simulink model "linearized_coupled_model"  (R2016b)
settings: Solver=VariableStepAuto  StartTime=0.0  StopTime=10.0  RelTol=1e-3
values from neighbouring files (symbols this model uses):
  A = simplify(A)    [symbolic_rotor.m]
  B_here = B_dbth    [riccati_controller_linear.m]
  C = [0,0,0,-L*mg*cos(beta)*beta_dot;0,0,0,L*mg*sin(beta)*beta_dot;0,0,0,0;0,0,0,0]    [disturbance_compensation_nonlinear_test.m]    (also in symbolic_rotor.m = [1,0,0,0, 0,0,0,0; uav_grasp_opt.m = [0,0,L*mg*sin(theta)*theta_dot;0,0,L*mg*cos(theta)*theta_dot; uav_grasp_opt_var_mass.m)
  K = diag([512,9,16])    [decoupling_falb_wolovich.m]
  V = inv(C*((B_here*K-A)\B_here))    [riccati_controller_linear.m]
  x0 = zeros(8,1)    [decoupling_falb_wolovich.m]    (also in disturbance_compensation.m; disturbance_compensation_nonlinear_test.m = [0;0;0;pi/2;0;0;0;0]; riccati_controller_linear.m; symbolic_rotor.m)
settings Model: Creator=Administrator  LastModifiedBy=Administrator

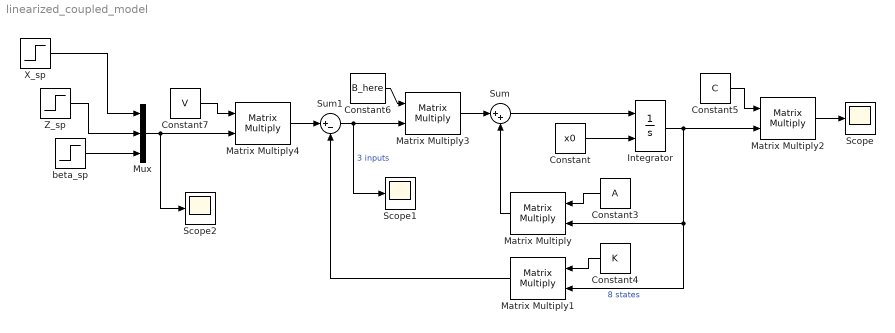
== system linearized_coupled_model ==
  Constant : Constant  Value=x0
  Constant3 : Constant  Value=A
  Constant4 : Constant  Value=K
  Constant5 : Constant  Value=C
  Constant6 : Constant  Value=B_here
  Constant7 : Constant  Value=V
  Integrator : Integrator  InitialConditionSource=external
  Matrix Multiply{,1..4} (5 alike) : Product  Multiplication=Matrix(*)
  Mux : Mux  Inputs=3
  Scope : Scope
  Scope1 : Scope
  Scope2 : Scope
  Sum : Sum  Inputs=|++
  Sum1 : Sum  Inputs=|+-
  X_sp : Step  SampleTime=0  VectorParams1D=off
  Z_sp : Step  SampleTime=0  VectorParams1D=off
  beta_sp : Step  Time=6  After=0.3  SampleTime=0  VectorParams1D=off
  wires:
  Constant/1 -> Integrator/2
  Sum/1 -> Integrator/1
  Integrator/1 -> Matrix Multiply1/2, Matrix Multiply/2, Matrix Multiply2/2  "8 states"
  Matrix Multiply/1 -> Sum/2
  Matrix Multiply3/1 -> Sum/1
  Matrix Multiply1/1 -> Sum1/2
  Matrix Multiply4/1 -> Sum1/1
  Matrix Multiply2/1 -> Scope/1
  Constant3/1 -> Matrix Multiply/1
  Mux/1 -> Scope2/1, Matrix Multiply4/2
  Constant7/1 -> Matrix Multiply4/1
  Constant6/1 -> Matrix Multiply3/1
  Sum1/1 -> Scope1/1, Matrix Multiply3/2  "3 inputs"
  Constant4/1 -> Matrix Multiply1/1
  Constant5/1 -> Matrix Multiply2/1
  X_sp/1 -> Mux/1
  Z_sp/1 -> Mux/2
  beta_sp/1 -> Mux/3
